simulink model "probable_final_fuzzy"  (R2021a)
settings: Solver=VariableStepAuto  StartTime=0.0  StopTime=720  RelTol=1e-3
undefined symbols (not defined in the file or in its folder): sigbuilder_block
libraries: fuzblock x2
settings Model: Creator=uddin  LastModifiedBy=uddin

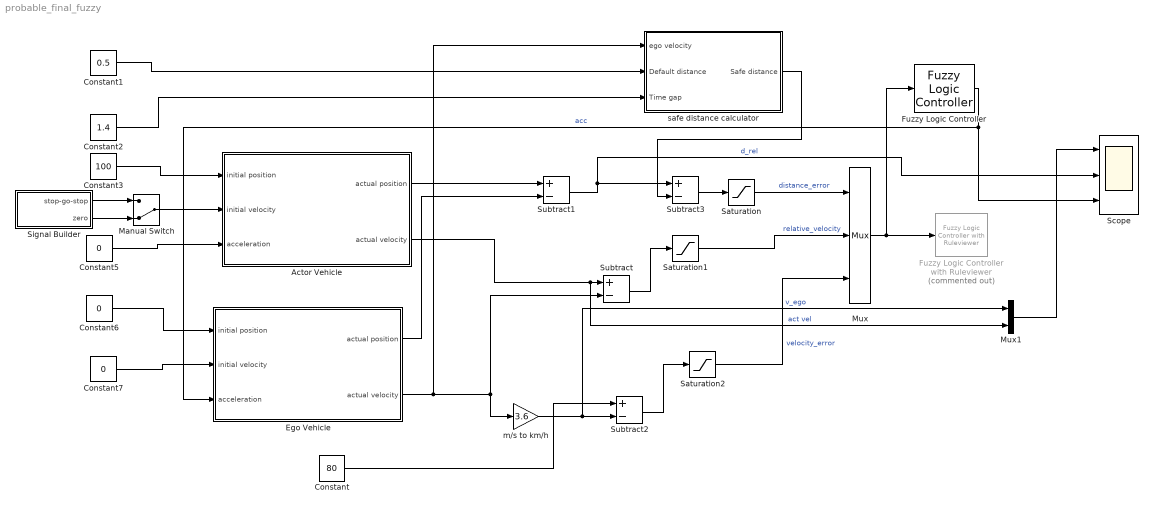
== system probable_final_fuzzy ==
  Actor Vehicle : Subsystem
  Constant : Constant  Value=80  SampleTime=1
  Constant1 : Constant  Value=0.5  SampleTime=1
  Constant2 : Constant  Value=1.4  SampleTime=1
  Constant3 : Constant  Value=100  SampleTime=1
  Constant5 : Constant  Value=0  SampleTime=1
  Constant6 : Constant  Value=0  SampleTime=1
  Constant7 : Constant  Value=0  SampleTime=1
  Ego Vehicle : Subsystem
  Fuzzy Logic Controller : fuzblock/Fuzzy Logic  Controller  FIS=self_created2  OutputSampleNumber=101  DataType=double  FuzzifiedInputs=off  RuleFiringStrengths=off  RuleOutputs=off  AggregatedOutputs=off  SimulateUsing=Interpreted execution  OutOfRangeInputValueMessage=none  NoRuleFiredMessage=none  EmptyOutputFuzzySetMessage=none
  Fuzzy Logic Controller with Ruleviewer : fuzblock/Fuzzy Logic  Controller  with Ruleviewer  Commented=on  fismatrix=self_created  Ts=2
  Manual Switch : ManualSwitch  CurrentSetting=0
  Mux : Mux  Inputs=3
  Mux1 : Mux  Inputs=2
  Saturation : Saturate  UpperLimit=1  LowerLimit=-1  LinearizeAsGain=off  ZeroCross=off
  Saturation1 : Saturate  UpperLimit=1  LowerLimit=-1  LinearizeAsGain=off  ZeroCross=off
  Saturation2 : Saturate  UpperLimit=1  LowerLimit=-1  LinearizeAsGain=off  ZeroCross=off
  Scope : Scope  NumInputPorts=3
  Signal Builder : Subsystem  Tag=STV Subsys  LoadFcn=sigbuilder_block('load');  StartFcn=sigbuilder_block('start');  StopFcn=sigbuilder_block('stop');  ClipboardFcn=sigbuilder_block('clipboard');  mask(Sigbuilder block){tuvar=[0:10]}
      mask help: Simulink:masks:SigbuilderBlock_MD
      mask init:
      | if ~strcmp(get_param(bdroot(gcbh),'SimulationStatus'),'stopped') tuvar = sigbuilder_block('maskInit'); end
      settings: CopyFcn=sigbuilder_block('copy');  DeleteFcn=sigbuilder_block('delete');  ModelCloseFcn=sigbuilder_block('modelClose');  PreSaveFcn=sigbuilder_block('preSave');  PauseFcn=sigbuilder_block('pause');  ContinueFcn=sigbuilder_block('continue');  NameChangeFcn=sigbuilder_block('namechange');  OpenFcn=sigbuilder_block('open',[393 134.4 550.8 400.2 ]);  CloseFcn=sigbuilder_block('close');
      mask Display: plot(0, 0, 100, 100,[2, 2, 32, 32, 2], [68, 8, 8, 68, 68],[32, 2], [38, 38], [32, 19, 2],[53, 60, 44], [32, 17, 17, 2],[16, 16, 31, 31]);txt = getActiveGroup(gcbh);text(2, 100, txt,'verticalAlignment', 'top');
  Subtract{,1..3} (4 alike) : Sum  Inputs=+-
  m/s to km/h : Gain  Gain=3.6
  safe distance calculator : Subsystem
  wires:
  Actor Vehicle/2(actual velocity) -> Mux1/2, Subtract/1  "act vel"
  Ego Vehicle/2(actual velocity) -> safe distance calculator/1(ego velocity), m/s to km/h/1, Subtract/2
  Actor Vehicle/1(actual position) -> Subtract1/1
  Ego Vehicle/1(actual position) -> Subtract1/2
  Subtract1/1 -> Scope/2, Subtract3/1  "d_rel"
  safe distance calculator/1(Safe distance) -> Subtract3/2
  Constant1/1 -> safe distance calculator/2(Default distance)
  Constant2/1 -> safe distance calculator/3(Time gap)
  Constant3/1 -> Actor Vehicle/1(initial position)
  Constant5/1 -> Actor Vehicle/3(acceleration)
  Constant6/1 -> Ego Vehicle/1(initial position)
  Constant7/1 -> Ego Vehicle/2(initial velocity)
  Subtract3/1 -> Saturation/1
  Subtract/1 -> Saturation1/1
  Subtract2/1 -> Saturation2/1
  Mux/1 -> Fuzzy Logic Controller/1, Fuzzy Logic Controller with Ruleviewer/1
  Saturation2/1 -> Mux/3  "velocity_error"
  Saturation1/1 -> Mux/2  "relative_velocity"
  Saturation/1 -> Mux/1  "distance_error"
  m/s to km/h/1 -> Mux1/1, Subtract2/2  "v_ego"
  Constant/1 -> Subtract2/1
  Fuzzy Logic Controller/1 -> Scope/3, Ego Vehicle/3(acceleration)  "acc"
  Mux1/1 -> Scope/1
  Signal Builder/1(stop-go-stop) -> Manual Switch/1
  Signal Builder/2(zero) -> Manual Switch/2
  Manual Switch/1 -> Actor Vehicle/2(initial velocity)

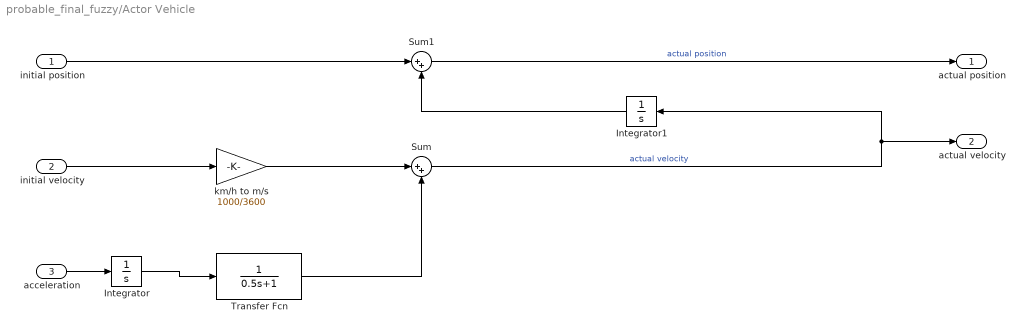
== system probable_final_fuzzy/Actor Vehicle ==
  initial position : Inport
  initial velocity : Inport  Port=2
  acceleration : Inport  Port=3
  Integrator : Integrator  ZeroCross=off
  Integrator1 : Integrator  ZeroCross=off
  Sum : Sum  Inputs=|++
  Sum1 : Sum  Inputs=|++
  Transfer Fcn : TransferFcn  Denominator=[0.5 1]
  km/h to m/s : Gain  Gain=1000/3600
  actual position : Outport
  actual velocity : Outport  Port=2
  wires:
  km/h to m/s/1 -> Sum/1
  initial velocity/1 -> km/h to m/s/1
  Transfer Fcn/1 -> Sum/2
  Integrator/1 -> Transfer Fcn/1
  Integrator1/1 -> Sum1/2
  initial position/1 -> Sum1/1
  acceleration/1 -> Integrator/1
  Sum/1 -> Integrator1/1, actual velocity/1  "actual velocity"
  Sum1/1 -> actual position/1  "actual position"

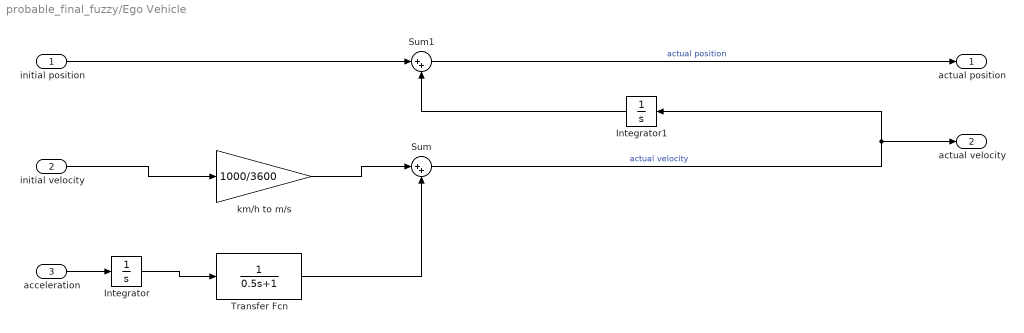
== system probable_final_fuzzy/Ego Vehicle ==
  initial position : Inport
  initial velocity : Inport  Port=2
  acceleration : Inport  Port=3
  Integrator : Integrator  ZeroCross=off
  Integrator1 : Integrator  ZeroCross=off
  Sum : Sum  Inputs=|++
  Sum1 : Sum  Inputs=|++
  Transfer Fcn : TransferFcn  Denominator=[0.5 1]
  km/h to m/s : Gain  Gain=1000/3600
  actual position : Outport
  actual velocity : Outport  Port=2
  wires:
  Sum1/1 -> actual position/1  "actual position"
  Sum/1 -> actual velocity/1, Integrator1/1  "actual velocity"
  acceleration/1 -> Integrator/1
  initial position/1 -> Sum1/1
  Integrator1/1 -> Sum1/2
  Integrator/1 -> Transfer Fcn/1
  Transfer Fcn/1 -> Sum/2
  initial velocity/1 -> km/h to m/s/1
  km/h to m/s/1 -> Sum/1

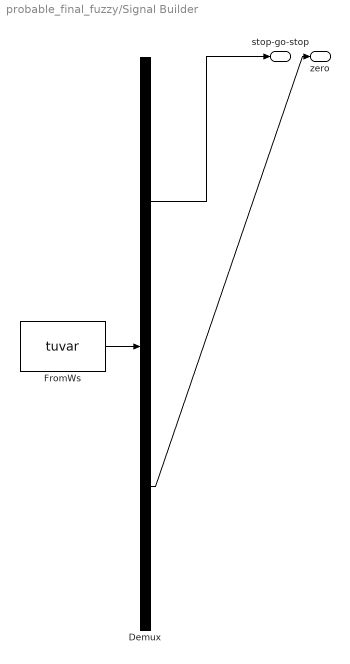
== system probable_final_fuzzy/Signal Builder ==
  Demux : Demux  Tag=STV Demux  Outputs=2
      settings: DisplayOption=none
  FromWs : FromWorkspace  Tag=STV FromWs  VariableName=tuvar
      SigBuilderData=|
      | common.afterFinalStr = 'Extrapolate'
      | common.sampleTime = 0
      | dataSet.timeRange = [0 30]
      | dataSet.name = 'Group 1'
      | sbobj.Groups.Name = 'Group 1'
      | sbobj.Groups.Signals(1).Name = 'stop-go-stop'
      | sbobj.Groups.Signals(1).XData = [0 5 10 20 25 30]
      | sbobj.Groups.Signals(1).YData = [0 0 2 2 0 0]
      | sbobj.Groups.Signals(2).Name = 'zero'
      | sbobj.Groups.Signals(2).XData = [0 30]
      | sbobj.Groups.Signals(2).YData = [0 0]
      | sbobj.Groups.TimeRange = [0 30]
  stop-go-stop : Outport  Tag=STV Outport
  zero : Outport  Tag=STV Outport  Port=2
  wires:
  FromWs/1 -> Demux/1
  Demux/1 -> stop-go-stop/1
  Demux/2 -> zero/1

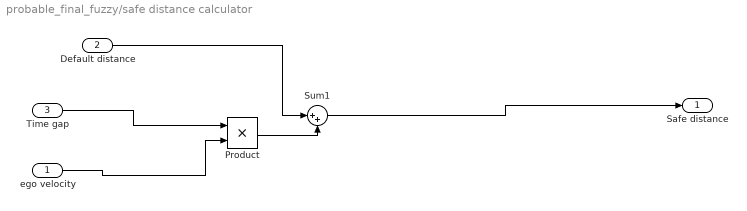
== system probable_final_fuzzy/safe distance calculator ==
  ego velocity : Inport
  Default distance : Inport  Port=2
  Time gap : Inport  Port=3
  Product : Product
  Sum1 : Sum  Inputs=|++
  Safe distance : Outport
  wires:
  Product/1 -> Sum1/2
  Sum1/1 -> Safe distance/1
  Time gap/1 -> Product/1
  Default distance/1 -> Sum1/1
  ego velocity/1 -> Product/2
